simulink model "ROPOD_Control_WheelsRL_Code_GEN"  (R2020b)
settings: Solver=VariableStepAuto  StartTime=0.0  StopTime=10.0  RelTol=1e-3
values from neighbouring files (symbols this model uses):
  FFtheta_intia = 0    [init_model.m]
  FFxy_mass = 0*80    (= 0)    [init_model.m]
  I_fhz_ddelta_cntr = 0    [init_model.m]
  I_fhz_dtheta_cntr = 0.3    [init_model.m]
  I_fhz_dxdy_cntr = 0.25    [init_model.m]
  K_gain_ddelta_cntr = 0.2    [init_model.m]
  K_gain_dtheta_cntr = 150    [init_model.m]
  K_gain_dxdy_cntr = 200    [init_model.m]
  LL_wp_fhz_ddelta_cntr = 10    [init_model.m]
  LL_wp_fhz_dtheta_cntr = 20    [init_model.m]
  LL_wp_fhz_dxdy_cntr = 20    [init_model.m]
  LL_wz_fhz_ddelta_cntr = 2    [init_model.m]
  LL_wz_fhz_dtheta_cntr = 20    [init_model.m]
  LL_wz_fhz_dxdy_cntr = 20    [init_model.m]
  LPF_fhz_ddelta_cntr = 10    [init_model.m]
  LPF_fhz_ddelta_meas = 50    [init_model.m]
  LPF_fhz_dtheta_cntr = 100    [init_model.m]
  LPF_fhz_dvarphi_meas = 50    [init_model.m]
  LPF_fhz_dxdy_cntr = 100    [init_model.m]
  max_hw_tau = 7.0    (= 7)    [init_model.m]
  max_ropod_acc_theta = 1.6    [init_model.m]
  max_ropod_acc_xy = 2.0    (= 2)    [init_model.m]
  max_ropod_sw_force = 500    [init_model.m]
  max_ropod_sw_tau = 250    [init_model.m]
  max_ropod_vel_theta = 1.6    [init_model.m]
  max_ropod_vel_xy = 2.0    (= 2)    [init_model.m]
  max_sw_current = 10    [init_model.m]
  Nwheels = 4    [Jqwl_numeric_function.m]    (also in S_matrix.m; extract_kinmodel_parameters.m; init_model.m; tau_optimal_dist_vec_fun.m)
  pivot_offs_sws = [3.835 3.465 2.059 0.357]    [init_model.m]
  ropod_kinmodel_pv = struct2array(ropod_kinmodel_param)    [set_ropod_KinModparams.m]
  SW_COM1_ENABLE1 = hex2dec('0001')    [init_model.m]
  SW_COM1_ENABLE2 = hex2dec('0002')    [init_model.m]
  SW_COM1_MODE_TORQUE = bitshift(hex2dec('0000'),2)    [init_model.m]
  SW_COM1_MODE_VELOCITY = bitshift(hex2dec('0002'),2)    [init_model.m]
  SW_COM1_USE_TS = hex2dec('8000')    [init_model.m]
  Tinit = 0*Tslot    [init_model.m]
  Ts = 0.001    [init_model.m]
undefined symbols (not defined in the file or in its folder): AgentNumber, DiscIntNeverNeededParam, flock_FFtheta_friction, flock_FFxy_friction, I_fhz_dtheta_flock_cntr, I_fhz_dvarphi_cntr, I_fhz_dxdy_flock_cntr, K_gain_dtheta_flock_cntr, K_gain_dvarphi_cntr, K_gain_dxdy_flock_cntr, LL_wp_fhz_dtheta_flock_cntr, LL_wp_fhz_dvarphi_cntr, LL_wp_fhz_dxdy_flock_cntr, LL_wz_fhz_dtheta_flock_cntr, LL_wz_fhz_dvarphi_cntr, LL_wz_fhz_dxdy_flock_cntr, LPF_fhz_dtheta_flock_cntr, LPF_fhz_dvarphi_cntr, LPF_fhz_dxdy_flock_cntr, max_flock_acc_theta, max_flock_acc_xy, max_flock_vel_theta, max_flock_vel_xy, Nagents, ropod_position_inflock, sw_tau_2_current, Tsflck
libraries: simulink x62, pid_lib x60, cstblocks x54, dspsigops x24, SOEM_EtherCAT_Lib x5, dspnetwork x4
(part 9 of 11)

== system ROPOD_Control_WheelsRL_Code_GEN/RopodTorqueDistribution_/pivot damping cntr/Pivot controller/G_I_LL_LPF Controller4/Shapeit Lead-Lag (Tustin) ==
  In : Inport
  fz : Inport  Port=2
  fp : Inport  Port=3
  Add : Sum  Inputs=+-
  Constant1 : Constant
  Constant2 : Constant  Value=0
  Constant4 : Constant
  Divide : Product  Inputs=*/
  Divide1 : Product  Inputs=/*
  Gain1 : Gain  Gain=2*pi
  Gain2 : Gain  Gain=2*pi
  PID Controller3 : pid_lib/PID Controller  Controller=PID  Form=Parallel  TimeDomain=Discrete-time  UseExternalTs=off  SampleTime=Ts  IntegratorMethod=Trapezoidal  FilterMethod=Trapezoidal  ControllerParametersSource=external  P=0.4  I=0.4*2*pi*3  D=0  UseFilter=on  N=100  TunerSelectOption=Transfer Function Based (PID Tuner App)  InitialConditionSource=internal  InitialConditionForIntegrator=0  InitialConditionForFilter=0  DifferentiatorICPrevScaledInput=0  ExternalReset=none  TrackingMode=off  Kt=1  LimitOutput=off  SatLimitsSource=internal  UpperSaturationLimit=max_hw_tau  LowerSaturationLimit=-max_hw_tau  LinearizeAsGain=on  AntiWindupMode=clamping  Kb=1  POutMin=[]  POutMax=[]  IOutMin=[]  IOutMax=[]  DOutMin=[]  DOutMax=[]  NOutMin=[]  NOutMax=[]  SumOutMin=[]  SumOutMax=[]  SaturationOutMin=[]  SaturationOutMax=[]  PParamMin=[]  PParamMax=[]  IParamMin=[]  IParamMax=[]  DParamMin=[]  DParamMax=[]  NParamMin=[]  NParamMax=[]  KbParamMin=[]  KbParamMax=[]  KtParamMin=[]  KtParamMax=[]  KbOutMin=[]  KbOutMax=[]  KtOutMin=[]  KtOutMax=[]  IntegratorOutMin=[]  IntegratorOutMax=[]  FilterOutMin=[]  FilterOutMax=[]  SumI1OutMin=[]  SumI1OutMax=[]  SumI2OutMin=[]  SumI2OutMax=[]  SumI3OutMin=[]  SumI3OutMax=[]  SumI4OutMin=[]  SumI4OutMax=[]  SumDOutMin=[]  SumDOutMax=[]  DifferentiatorOutMin=[]  DifferentiatorOutMax=[]  FilterDiffOutCoefMin=[]  FilterDiffOutCoefMax=[]  ReciprocalOutMin=[]  ReciprocalOutMax=[]  SumDenOutMin=[]  SumDenOutMax=[]  SumNumOutMin=[]  SumNumOutMax=[]  DivideOutMin=[]  DivideOutMax=[]  UdiffTsProdOutMin=[]  UdiffTsProdOutMax=[]  NTsProdOutMin=[]  NTsProdOutMax=[]  UintegralTsProdOutMin=[]  UintegralTsProdOutMax=[]  UngainTsProdOutMin=[]  UngainTsProdOutMax=[]  IntegratorContinuousStateAttributes=''  IntegratorStateMustResolveToSignalObject=off  IntegratorRTWStateStorageClass=Auto  FilterContinuousStateAttributes=''  FilterStateMustResolveToSignalObject=off  FilterRTWStateStorageClass=Auto  ParallelPVariant=ExternalParameters  IdealPVariant=Disabled  IVariant=ExternalParameters  DVariant=ExternalParameters  IntegratorVariant=Discrete  SatVariant=Disabled  AWVariant=Passthrough  PCopyVariant=Disabled  TRVariant=Disabled  FdbkBlocksVariant=Forward  IdealPFdbkVariant=Disabled  SatFdbkVariant=Disabled  DerivativeFilterVariant=TrapezoidalFilter  NVariant=ExternalParameters  NCopyVariant=ExternalParameters  FilterICVariant=InternalICsFilter  IntegratorICVariant=InternalICs  ExternalResetVariant=Disabled  TRSumVariant=Passthrough  SumFdbkVariant=Disabled  SumVariant=Sum_PID  TsampFilterVariant=InternalTs  TsampNgainVariant=Passthrough  TsampIntegralVariant=Passthrough  ExternalSaturationOutDataTypeStr=Inherit: Same as second input
  Out : Outport  VectorParamsAs1DForOutWhenUnconnected=off
  wires:
  Constant4/1 -> PID Controller3/2
  In/1 -> PID Controller3/1
  PID Controller3/1 -> Out/1
  fz/1 -> Gain2/1
  fp/1 -> Gain1/1
  Gain1/1 -> PID Controller3/5, Divide/2
  Constant2/1 -> PID Controller3/3
  Gain2/1 -> Divide1/1, Divide/1
  Divide/1 -> Add/2
  Constant1/1 -> Add/1
  Add/1 -> Divide1/2
  Divide1/1 -> PID Controller3/4

== system ROPOD_Control_WheelsRL_Code_GEN/RopodTorqueDistribution_/wheel vel cntr/Wheels Velocity controller/G_I_LL_LPF Controller1/Shapeit Integrator (Tustin) ==
  In : Inport
  I_fhz : Inport  Port=2
  reset : Inport  Port=3
  Constant : Constant  Value=0
  Constant4 : Constant
  Constant5 : Constant  Value=0
  Gain2 : Gain  Gain=2*pi
  PID Controller3 : pid_lib/PID Controller  Controller=PID  Form=Parallel  TimeDomain=Discrete-time  UseExternalTs=off  SampleTime=Ts  IntegratorMethod=Trapezoidal  FilterMethod=Trapezoidal  ControllerParametersSource=external  P=0.4  I=0.4*2*pi*3  D=0  UseFilter=on  N=100  TunerSelectOption=Transfer Function Based (PID Tuner App)  InitialConditionSource=internal  InitialConditionForIntegrator=0  InitialConditionForFilter=0  DifferentiatorICPrevScaledInput=0  ExternalReset=level  TrackingMode=off  Kt=1  LimitOutput=on  SatLimitsSource=internal  UpperSaturationLimit=max_hw_tau  LowerSaturationLimit=-max_hw_tau  LinearizeAsGain=on  AntiWindupMode=clamping  Kb=1  POutMin=[]  POutMax=[]  IOutMin=[]  IOutMax=[]  DOutMin=[]  DOutMax=[]  NOutMin=[]  NOutMax=[]  SumOutMin=[]  SumOutMax=[]  SaturationOutMin=[]  SaturationOutMax=[]  PParamMin=[]  PParamMax=[]  IParamMin=[]  IParamMax=[]  DParamMin=[]  DParamMax=[]  NParamMin=[]  NParamMax=[]  KbParamMin=[]  KbParamMax=[]  KtParamMin=[]  KtParamMax=[]  KbOutMin=[]  KbOutMax=[]  KtOutMin=[]  KtOutMax=[]  IntegratorOutMin=[]  IntegratorOutMax=[]  FilterOutMin=[]  FilterOutMax=[]  SumI1OutMin=[]  SumI1OutMax=[]  SumI2OutMin=[]  SumI2OutMax=[]  SumI3OutMin=[]  SumI3OutMax=[]  SumI4OutMin=[]  SumI4OutMax=[]  SumDOutMin=[]  SumDOutMax=[]  DifferentiatorOutMin=[]  DifferentiatorOutMax=[]  FilterDiffOutCoefMin=[]  FilterDiffOutCoefMax=[]  ReciprocalOutMin=[]  ReciprocalOutMax=[]  SumDenOutMin=[]  SumDenOutMax=[]  SumNumOutMin=[]  SumNumOutMax=[]  DivideOutMin=[]  DivideOutMax=[]  UdiffTsProdOutMin=[]  UdiffTsProdOutMax=[]  NTsProdOutMin=[]  NTsProdOutMax=[]  UintegralTsProdOutMin=[]  UintegralTsProdOutMax=[]  UngainTsProdOutMin=[]  UngainTsProdOutMax=[]  IntegratorContinuousStateAttributes=''  IntegratorStateMustResolveToSignalObject=off  IntegratorRTWStateStorageClass=Auto  FilterContinuousStateAttributes=''  FilterStateMustResolveToSignalObject=off  FilterRTWStateStorageClass=Auto  ParallelPVariant=ExternalParameters  IdealPVariant=Disabled  IVariant=ExternalParameters  DVariant=ExternalParameters  IntegratorVariant=Discrete  SatVariant=Enabled  AWVariant=DiscClampingParallel  PCopyVariant=Disabled  TRVariant=Disabled  FdbkBlocksVariant=Feedback  IdealPFdbkVariant=Passthrough  SatFdbkVariant=Passthrough  DerivativeFilterVariant=TrapezoidalFilter  NVariant=ExternalParameters  NCopyVariant=ExternalParameters  FilterICVariant=InternalICsFilter  IntegratorICVariant=InternalICs  ExternalResetVariant=ExternalReset  TRSumVariant=Passthrough  SumFdbkVariant=Enabled  SumVariant=Sum_PID  TsampFilterVariant=InternalTs  TsampNgainVariant=Passthrough  TsampIntegralVariant=Passthrough  ExternalSaturationOutDataTypeStr=Inherit: Same as second input
  Product4 : Product
  Out : Outport  VectorParamsAs1DForOutWhenUnconnected=off
  wires:
  I_fhz/1 -> Product4/2
  Product4/1 -> Gain2/1
  reset/1 -> PID Controller3/6
  Gain2/1 -> PID Controller3/3
  PID Controller3/1 -> Out/1
  In/1 -> PID Controller3/1
  Constant4/1 -> Product4/1, PID Controller3/2
  Constant5/1 -> PID Controller3/5
  Constant/1 -> PID Controller3/4

== system ROPOD_Control_WheelsRL_Code_GEN/RopodTorqueDistribution_/wheel vel cntr/Wheels Velocity controller/G_I_LL_LPF Controller1/Shapeit Lead-Lag (Tustin) ==
  In : Inport
  fz : Inport  Port=2
  fp : Inport  Port=3
  Add : Sum  Inputs=+-
  Constant1 : Constant
  Constant2 : Constant  Value=0
  Constant4 : Constant
  Divide : Product  Inputs=*/
  Divide1 : Product  Inputs=/*
  Gain1 : Gain  Gain=2*pi
  Gain2 : Gain  Gain=2*pi
  PID Controller3 : pid_lib/PID Controller  Controller=PID  Form=Parallel  TimeDomain=Discrete-time  UseExternalTs=off  SampleTime=Ts  IntegratorMethod=Trapezoidal  FilterMethod=Trapezoidal  ControllerParametersSource=external  P=0.4  I=0.4*2*pi*3  D=0  UseFilter=on  N=100  TunerSelectOption=Transfer Function Based (PID Tuner App)  InitialConditionSource=internal  InitialConditionForIntegrator=0  InitialConditionForFilter=0  DifferentiatorICPrevScaledInput=0  ExternalReset=none  TrackingMode=off  Kt=1  LimitOutput=off  SatLimitsSource=internal  UpperSaturationLimit=max_hw_tau  LowerSaturationLimit=-max_hw_tau  LinearizeAsGain=on  AntiWindupMode=clamping  Kb=1  POutMin=[]  POutMax=[]  IOutMin=[]  IOutMax=[]  DOutMin=[]  DOutMax=[]  NOutMin=[]  NOutMax=[]  SumOutMin=[]  SumOutMax=[]  SaturationOutMin=[]  SaturationOutMax=[]  PParamMin=[]  PParamMax=[]  IParamMin=[]  IParamMax=[]  DParamMin=[]  DParamMax=[]  NParamMin=[]  NParamMax=[]  KbParamMin=[]  KbParamMax=[]  KtParamMin=[]  KtParamMax=[]  KbOutMin=[]  KbOutMax=[]  KtOutMin=[]  KtOutMax=[]  IntegratorOutMin=[]  IntegratorOutMax=[]  FilterOutMin=[]  FilterOutMax=[]  SumI1OutMin=[]  SumI1OutMax=[]  SumI2OutMin=[]  SumI2OutMax=[]  SumI3OutMin=[]  SumI3OutMax=[]  SumI4OutMin=[]  SumI4OutMax=[]  SumDOutMin=[]  SumDOutMax=[]  DifferentiatorOutMin=[]  DifferentiatorOutMax=[]  FilterDiffOutCoefMin=[]  FilterDiffOutCoefMax=[]  ReciprocalOutMin=[]  ReciprocalOutMax=[]  SumDenOutMin=[]  SumDenOutMax=[]  SumNumOutMin=[]  SumNumOutMax=[]  DivideOutMin=[]  DivideOutMax=[]  UdiffTsProdOutMin=[]  UdiffTsProdOutMax=[]  NTsProdOutMin=[]  NTsProdOutMax=[]  UintegralTsProdOutMin=[]  UintegralTsProdOutMax=[]  UngainTsProdOutMin=[]  UngainTsProdOutMax=[]  IntegratorContinuousStateAttributes=''  IntegratorStateMustResolveToSignalObject=off  IntegratorRTWStateStorageClass=Auto  FilterContinuousStateAttributes=''  FilterStateMustResolveToSignalObject=off  FilterRTWStateStorageClass=Auto  ParallelPVariant=ExternalParameters  IdealPVariant=Disabled  IVariant=ExternalParameters  DVariant=ExternalParameters  IntegratorVariant=Discrete  SatVariant=Disabled  AWVariant=Passthrough  PCopyVariant=Disabled  TRVariant=Disabled  FdbkBlocksVariant=Forward  IdealPFdbkVariant=Disabled  SatFdbkVariant=Disabled  DerivativeFilterVariant=TrapezoidalFilter  NVariant=ExternalParameters  NCopyVariant=ExternalParameters  FilterICVariant=InternalICsFilter  IntegratorICVariant=InternalICs  ExternalResetVariant=Disabled  TRSumVariant=Passthrough  SumFdbkVariant=Disabled  SumVariant=Sum_PID  TsampFilterVariant=InternalTs  TsampNgainVariant=Passthrough  TsampIntegralVariant=Passthrough  ExternalSaturationOutDataTypeStr=Inherit: Same as second input
  Out : Outport  VectorParamsAs1DForOutWhenUnconnected=off
  wires:
  Constant4/1 -> PID Controller3/2
  In/1 -> PID Controller3/1
  PID Controller3/1 -> Out/1
  fz/1 -> Gain2/1
  fp/1 -> Gain1/1
  Gain1/1 -> PID Controller3/5, Divide/2
  Constant2/1 -> PID Controller3/3
  Gain2/1 -> Divide1/1, Divide/1
  Divide/1 -> Add/2
  Constant1/1 -> Add/1
  Add/1 -> Divide1/2
  Divide1/1 -> PID Controller3/4

== system ROPOD_Control_WheelsRL_Code_GEN/RopodTorqueDistribution_/wheel vel cntr/Wheels Velocity controller/G_I_LL_LPF Controller2/Shapeit Integrator (Tustin) ==
  In : Inport
  I_fhz : Inport  Port=2
  reset : Inport  Port=3
  Constant : Constant  Value=0
  Constant4 : Constant
  Constant5 : Constant  Value=0
  Gain2 : Gain  Gain=2*pi
  PID Controller3 : pid_lib/PID Controller  Controller=PID  Form=Parallel  TimeDomain=Discrete-time  UseExternalTs=off  SampleTime=Ts  IntegratorMethod=Trapezoidal  FilterMethod=Trapezoidal  ControllerParametersSource=external  P=0.4  I=0.4*2*pi*3  D=0  UseFilter=on  N=100  TunerSelectOption=Transfer Function Based (PID Tuner App)  InitialConditionSource=internal  InitialConditionForIntegrator=0  InitialConditionForFilter=0  DifferentiatorICPrevScaledInput=0  ExternalReset=level  TrackingMode=off  Kt=1  LimitOutput=on  SatLimitsSource=internal  UpperSaturationLimit=max_hw_tau  LowerSaturationLimit=-max_hw_tau  LinearizeAsGain=on  AntiWindupMode=clamping  Kb=1  POutMin=[]  POutMax=[]  IOutMin=[]  IOutMax=[]  DOutMin=[]  DOutMax=[]  NOutMin=[]  NOutMax=[]  SumOutMin=[]  SumOutMax=[]  SaturationOutMin=[]  SaturationOutMax=[]  PParamMin=[]  PParamMax=[]  IParamMin=[]  IParamMax=[]  DParamMin=[]  DParamMax=[]  NParamMin=[]  NParamMax=[]  KbParamMin=[]  KbParamMax=[]  KtParamMin=[]  KtParamMax=[]  KbOutMin=[]  KbOutMax=[]  KtOutMin=[]  KtOutMax=[]  IntegratorOutMin=[]  IntegratorOutMax=[]  FilterOutMin=[]  FilterOutMax=[]  SumI1OutMin=[]  SumI1OutMax=[]  SumI2OutMin=[]  SumI2OutMax=[]  SumI3OutMin=[]  SumI3OutMax=[]  SumI4OutMin=[]  SumI4OutMax=[]  SumDOutMin=[]  SumDOutMax=[]  DifferentiatorOutMin=[]  DifferentiatorOutMax=[]  FilterDiffOutCoefMin=[]  FilterDiffOutCoefMax=[]  ReciprocalOutMin=[]  ReciprocalOutMax=[]  SumDenOutMin=[]  SumDenOutMax=[]  SumNumOutMin=[]  SumNumOutMax=[]  DivideOutMin=[]  DivideOutMax=[]  UdiffTsProdOutMin=[]  UdiffTsProdOutMax=[]  NTsProdOutMin=[]  NTsProdOutMax=[]  UintegralTsProdOutMin=[]  UintegralTsProdOutMax=[]  UngainTsProdOutMin=[]  UngainTsProdOutMax=[]  IntegratorContinuousStateAttributes=''  IntegratorStateMustResolveToSignalObject=off  IntegratorRTWStateStorageClass=Auto  FilterContinuousStateAttributes=''  FilterStateMustResolveToSignalObject=off  FilterRTWStateStorageClass=Auto  ParallelPVariant=ExternalParameters  IdealPVariant=Disabled  IVariant=ExternalParameters  DVariant=ExternalParameters  IntegratorVariant=Discrete  SatVariant=Enabled  AWVariant=DiscClampingParallel  PCopyVariant=Disabled  TRVariant=Disabled  FdbkBlocksVariant=Feedback  IdealPFdbkVariant=Passthrough  SatFdbkVariant=Passthrough  DerivativeFilterVariant=TrapezoidalFilter  NVariant=ExternalParameters  NCopyVariant=ExternalParameters  FilterICVariant=InternalICsFilter  IntegratorICVariant=InternalICs  ExternalResetVariant=ExternalReset  TRSumVariant=Passthrough  SumFdbkVariant=Enabled  SumVariant=Sum_PID  TsampFilterVariant=InternalTs  TsampNgainVariant=Passthrough  TsampIntegralVariant=Passthrough  ExternalSaturationOutDataTypeStr=Inherit: Same as second input
  Product4 : Product
  Out : Outport  VectorParamsAs1DForOutWhenUnconnected=off
  wires:
  I_fhz/1 -> Product4/2
  Product4/1 -> Gain2/1
  reset/1 -> PID Controller3/6
  Gain2/1 -> PID Controller3/3
  PID Controller3/1 -> Out/1
  In/1 -> PID Controller3/1
  Constant4/1 -> Product4/1, PID Controller3/2
  Constant5/1 -> PID Controller3/5
  Constant/1 -> PID Controller3/4

== system ROPOD_Control_WheelsRL_Code_GEN/RopodTorqueDistribution_/wheel vel cntr/Wheels Velocity controller/G_I_LL_LPF Controller2/Shapeit Lead-Lag (Tustin) ==
  In : Inport
  fz : Inport  Port=2
  fp : Inport  Port=3
  Add : Sum  Inputs=+-
  Constant1 : Constant
  Constant2 : Constant  Value=0
  Constant4 : Constant
  Divide : Product  Inputs=*/
  Divide1 : Product  Inputs=/*
  Gain1 : Gain  Gain=2*pi
  Gain2 : Gain  Gain=2*pi
  PID Controller3 : pid_lib/PID Controller  Controller=PID  Form=Parallel  TimeDomain=Discrete-time  UseExternalTs=off  SampleTime=Ts  IntegratorMethod=Trapezoidal  FilterMethod=Trapezoidal  ControllerParametersSource=external  P=0.4  I=0.4*2*pi*3  D=0  UseFilter=on  N=100  TunerSelectOption=Transfer Function Based (PID Tuner App)  InitialConditionSource=internal  InitialConditionForIntegrator=0  InitialConditionForFilter=0  DifferentiatorICPrevScaledInput=0  ExternalReset=none  TrackingMode=off  Kt=1  LimitOutput=off  SatLimitsSource=internal  UpperSaturationLimit=max_hw_tau  LowerSaturationLimit=-max_hw_tau  LinearizeAsGain=on  AntiWindupMode=clamping  Kb=1  POutMin=[]  POutMax=[]  IOutMin=[]  IOutMax=[]  DOutMin=[]  DOutMax=[]  NOutMin=[]  NOutMax=[]  SumOutMin=[]  SumOutMax=[]  SaturationOutMin=[]  SaturationOutMax=[]  PParamMin=[]  PParamMax=[]  IParamMin=[]  IParamMax=[]  DParamMin=[]  DParamMax=[]  NParamMin=[]  NParamMax=[]  KbParamMin=[]  KbParamMax=[]  KtParamMin=[]  KtParamMax=[]  KbOutMin=[]  KbOutMax=[]  KtOutMin=[]  KtOutMax=[]  IntegratorOutMin=[]  IntegratorOutMax=[]  FilterOutMin=[]  FilterOutMax=[]  SumI1OutMin=[]  SumI1OutMax=[]  SumI2OutMin=[]  SumI2OutMax=[]  SumI3OutMin=[]  SumI3OutMax=[]  SumI4OutMin=[]  SumI4OutMax=[]  SumDOutMin=[]  SumDOutMax=[]  DifferentiatorOutMin=[]  DifferentiatorOutMax=[]  FilterDiffOutCoefMin=[]  FilterDiffOutCoefMax=[]  ReciprocalOutMin=[]  ReciprocalOutMax=[]  SumDenOutMin=[]  SumDenOutMax=[]  SumNumOutMin=[]  SumNumOutMax=[]  DivideOutMin=[]  DivideOutMax=[]  UdiffTsProdOutMin=[]  UdiffTsProdOutMax=[]  NTsProdOutMin=[]  NTsProdOutMax=[]  UintegralTsProdOutMin=[]  UintegralTsProdOutMax=[]  UngainTsProdOutMin=[]  UngainTsProdOutMax=[]  IntegratorContinuousStateAttributes=''  IntegratorStateMustResolveToSignalObject=off  IntegratorRTWStateStorageClass=Auto  FilterContinuousStateAttributes=''  FilterStateMustResolveToSignalObject=off  FilterRTWStateStorageClass=Auto  ParallelPVariant=ExternalParameters  IdealPVariant=Disabled  IVariant=ExternalParameters  DVariant=ExternalParameters  IntegratorVariant=Discrete  SatVariant=Disabled  AWVariant=Passthrough  PCopyVariant=Disabled  TRVariant=Disabled  FdbkBlocksVariant=Forward  IdealPFdbkVariant=Disabled  SatFdbkVariant=Disabled  DerivativeFilterVariant=TrapezoidalFilter  NVariant=ExternalParameters  NCopyVariant=ExternalParameters  FilterICVariant=InternalICsFilter  IntegratorICVariant=InternalICs  ExternalResetVariant=Disabled  TRSumVariant=Passthrough  SumFdbkVariant=Disabled  SumVariant=Sum_PID  TsampFilterVariant=InternalTs  TsampNgainVariant=Passthrough  TsampIntegralVariant=Passthrough  ExternalSaturationOutDataTypeStr=Inherit: Same as second input
  Out : Outport  VectorParamsAs1DForOutWhenUnconnected=off
  wires:
  Constant4/1 -> PID Controller3/2
  In/1 -> PID Controller3/1
  PID Controller3/1 -> Out/1
  fz/1 -> Gain2/1
  fp/1 -> Gain1/1
  Gain1/1 -> PID Controller3/5, Divide/2
  Constant2/1 -> PID Controller3/3
  Gain2/1 -> Divide1/1, Divide/1
  Divide/1 -> Add/2
  Constant1/1 -> Add/1
  Add/1 -> Divide1/2
  Divide1/1 -> PID Controller3/4

== system ROPOD_Control_WheelsRL_Code_GEN/RopodTorqueDistribution_/wheel vel cntr/Wheels Velocity controller/G_I_LL_LPF Controller3/Shapeit Integrator (Tustin) ==
  In : Inport
  I_fhz : Inport  Port=2
  reset : Inport  Port=3
  Constant : Constant  Value=0
  Constant4 : Constant
  Constant5 : Constant  Value=0
  Gain2 : Gain  Gain=2*pi
  PID Controller3 : pid_lib/PID Controller  Controller=PID  Form=Parallel  TimeDomain=Discrete-time  UseExternalTs=off  SampleTime=Ts  IntegratorMethod=Trapezoidal  FilterMethod=Trapezoidal  ControllerParametersSource=external  P=0.4  I=0.4*2*pi*3  D=0  UseFilter=on  N=100  TunerSelectOption=Transfer Function Based (PID Tuner App)  InitialConditionSource=internal  InitialConditionForIntegrator=0  InitialConditionForFilter=0  DifferentiatorICPrevScaledInput=0  ExternalReset=level  TrackingMode=off  Kt=1  LimitOutput=on  SatLimitsSource=internal  UpperSaturationLimit=max_hw_tau  LowerSaturationLimit=-max_hw_tau  LinearizeAsGain=on  AntiWindupMode=clamping  Kb=1  POutMin=[]  POutMax=[]  IOutMin=[]  IOutMax=[]  DOutMin=[]  DOutMax=[]  NOutMin=[]  NOutMax=[]  SumOutMin=[]  SumOutMax=[]  SaturationOutMin=[]  SaturationOutMax=[]  PParamMin=[]  PParamMax=[]  IParamMin=[]  IParamMax=[]  DParamMin=[]  DParamMax=[]  NParamMin=[]  NParamMax=[]  KbParamMin=[]  KbParamMax=[]  KtParamMin=[]  KtParamMax=[]  KbOutMin=[]  KbOutMax=[]  KtOutMin=[]  KtOutMax=[]  IntegratorOutMin=[]  IntegratorOutMax=[]  FilterOutMin=[]  FilterOutMax=[]  SumI1OutMin=[]  SumI1OutMax=[]  SumI2OutMin=[]  SumI2OutMax=[]  SumI3OutMin=[]  SumI3OutMax=[]  SumI4OutMin=[]  SumI4OutMax=[]  SumDOutMin=[]  SumDOutMax=[]  DifferentiatorOutMin=[]  DifferentiatorOutMax=[]  FilterDiffOutCoefMin=[]  FilterDiffOutCoefMax=[]  ReciprocalOutMin=[]  ReciprocalOutMax=[]  SumDenOutMin=[]  SumDenOutMax=[]  SumNumOutMin=[]  SumNumOutMax=[]  DivideOutMin=[]  DivideOutMax=[]  UdiffTsProdOutMin=[]  UdiffTsProdOutMax=[]  NTsProdOutMin=[]  NTsProdOutMax=[]  UintegralTsProdOutMin=[]  UintegralTsProdOutMax=[]  UngainTsProdOutMin=[]  UngainTsProdOutMax=[]  IntegratorContinuousStateAttributes=''  IntegratorStateMustResolveToSignalObject=off  IntegratorRTWStateStorageClass=Auto  FilterContinuousStateAttributes=''  FilterStateMustResolveToSignalObject=off  FilterRTWStateStorageClass=Auto  ParallelPVariant=ExternalParameters  IdealPVariant=Disabled  IVariant=ExternalParameters  DVariant=ExternalParameters  IntegratorVariant=Discrete  SatVariant=Enabled  AWVariant=DiscClampingParallel  PCopyVariant=Disabled  TRVariant=Disabled  FdbkBlocksVariant=Feedback  IdealPFdbkVariant=Passthrough  SatFdbkVariant=Passthrough  DerivativeFilterVariant=TrapezoidalFilter  NVariant=ExternalParameters  NCopyVariant=ExternalParameters  FilterICVariant=InternalICsFilter  IntegratorICVariant=InternalICs  ExternalResetVariant=ExternalReset  TRSumVariant=Passthrough  SumFdbkVariant=Enabled  SumVariant=Sum_PID  TsampFilterVariant=InternalTs  TsampNgainVariant=Passthrough  TsampIntegralVariant=Passthrough  ExternalSaturationOutDataTypeStr=Inherit: Same as second input
  Product4 : Product
  Out : Outport  VectorParamsAs1DForOutWhenUnconnected=off
  wires:
  Constant/1 -> PID Controller3/4
  Constant5/1 -> PID Controller3/5
  Constant4/1 -> PID Controller3/2, Product4/1
  In/1 -> PID Controller3/1
  PID Controller3/1 -> Out/1
  Gain2/1 -> PID Controller3/3
  reset/1 -> PID Controller3/6
  Product4/1 -> Gain2/1
  I_fhz/1 -> Product4/2

== system ROPOD_Control_WheelsRL_Code_GEN/RopodTorqueDistribution_/wheel vel cntr/Wheels Velocity controller/G_I_LL_LPF Controller3/Shapeit Lead-Lag (Tustin) ==
  In : Inport
  fz : Inport  Port=2
  fp : Inport  Port=3
  Add : Sum  Inputs=+-
  Constant1 : Constant
  Constant2 : Constant  Value=0
  Constant4 : Constant
  Divide : Product  Inputs=*/
  Divide1 : Product  Inputs=/*
  Gain1 : Gain  Gain=2*pi
  Gain2 : Gain  Gain=2*pi
  PID Controller3 : pid_lib/PID Controller  Controller=PID  Form=Parallel  TimeDomain=Discrete-time  UseExternalTs=off  SampleTime=Ts  IntegratorMethod=Trapezoidal  FilterMethod=Trapezoidal  ControllerParametersSource=external  P=0.4  I=0.4*2*pi*3  D=0  UseFilter=on  N=100  TunerSelectOption=Transfer Function Based (PID Tuner App)  InitialConditionSource=internal  InitialConditionForIntegrator=0  InitialConditionForFilter=0  DifferentiatorICPrevScaledInput=0  ExternalReset=none  TrackingMode=off  Kt=1  LimitOutput=off  SatLimitsSource=internal  UpperSaturationLimit=max_hw_tau  LowerSaturationLimit=-max_hw_tau  LinearizeAsGain=on  AntiWindupMode=clamping  Kb=1  POutMin=[]  POutMax=[]  IOutMin=[]  IOutMax=[]  DOutMin=[]  DOutMax=[]  NOutMin=[]  NOutMax=[]  SumOutMin=[]  SumOutMax=[]  SaturationOutMin=[]  SaturationOutMax=[]  PParamMin=[]  PParamMax=[]  IParamMin=[]  IParamMax=[]  DParamMin=[]  DParamMax=[]  NParamMin=[]  NParamMax=[]  KbParamMin=[]  KbParamMax=[]  KtParamMin=[]  KtParamMax=[]  KbOutMin=[]  KbOutMax=[]  KtOutMin=[]  KtOutMax=[]  IntegratorOutMin=[]  IntegratorOutMax=[]  FilterOutMin=[]  FilterOutMax=[]  SumI1OutMin=[]  SumI1OutMax=[]  SumI2OutMin=[]  SumI2OutMax=[]  SumI3OutMin=[]  SumI3OutMax=[]  SumI4OutMin=[]  SumI4OutMax=[]  SumDOutMin=[]  SumDOutMax=[]  DifferentiatorOutMin=[]  DifferentiatorOutMax=[]  FilterDiffOutCoefMin=[]  FilterDiffOutCoefMax=[]  ReciprocalOutMin=[]  ReciprocalOutMax=[]  SumDenOutMin=[]  SumDenOutMax=[]  SumNumOutMin=[]  SumNumOutMax=[]  DivideOutMin=[]  DivideOutMax=[]  UdiffTsProdOutMin=[]  UdiffTsProdOutMax=[]  NTsProdOutMin=[]  NTsProdOutMax=[]  UintegralTsProdOutMin=[]  UintegralTsProdOutMax=[]  UngainTsProdOutMin=[]  UngainTsProdOutMax=[]  IntegratorContinuousStateAttributes=''  IntegratorStateMustResolveToSignalObject=off  IntegratorRTWStateStorageClass=Auto  FilterContinuousStateAttributes=''  FilterStateMustResolveToSignalObject=off  FilterRTWStateStorageClass=Auto  ParallelPVariant=ExternalParameters  IdealPVariant=Disabled  IVariant=ExternalParameters  DVariant=ExternalParameters  IntegratorVariant=Discrete  SatVariant=Disabled  AWVariant=Passthrough  PCopyVariant=Disabled  TRVariant=Disabled  FdbkBlocksVariant=Forward  IdealPFdbkVariant=Disabled  SatFdbkVariant=Disabled  DerivativeFilterVariant=TrapezoidalFilter  NVariant=ExternalParameters  NCopyVariant=ExternalParameters  FilterICVariant=InternalICsFilter  IntegratorICVariant=InternalICs  ExternalResetVariant=Disabled  TRSumVariant=Passthrough  SumFdbkVariant=Disabled  SumVariant=Sum_PID  TsampFilterVariant=InternalTs  TsampNgainVariant=Passthrough  TsampIntegralVariant=Passthrough  ExternalSaturationOutDataTypeStr=Inherit: Same as second input
  Out : Outport  VectorParamsAs1DForOutWhenUnconnected=off
  wires:
  Divide1/1 -> PID Controller3/4
  Add/1 -> Divide1/2
  Constant1/1 -> Add/1
  Divide/1 -> Add/2
  Gain2/1 -> Divide/1, Divide1/1
  Constant2/1 -> PID Controller3/3
  Gain1/1 -> Divide/2, PID Controller3/5
  fp/1 -> Gain1/1
  fz/1 -> Gain2/1
  PID Controller3/1 -> Out/1
  In/1 -> PID Controller3/1
  Constant4/1 -> PID Controller3/2

== system ROPOD_Control_WheelsRL_Code_GEN/RopodTorqueDistribution_/wheel vel cntr/Wheels Velocity controller/G_I_LL_LPF Controller4/Shapeit Integrator (Tustin) ==
  In : Inport
  I_fhz : Inport  Port=2
  reset : Inport  Port=3
  Constant : Constant  Value=0
  Constant4 : Constant
  Constant5 : Constant  Value=0
  Gain2 : Gain  Gain=2*pi
  PID Controller3 : pid_lib/PID Controller  Controller=PID  Form=Parallel  TimeDomain=Discrete-time  UseExternalTs=off  SampleTime=Ts  IntegratorMethod=Trapezoidal  FilterMethod=Trapezoidal  ControllerParametersSource=external  P=0.4  I=0.4*2*pi*3  D=0  UseFilter=on  N=100  TunerSelectOption=Transfer Function Based (PID Tuner App)  InitialConditionSource=internal  InitialConditionForIntegrator=0  InitialConditionForFilter=0  DifferentiatorICPrevScaledInput=0  ExternalReset=level  TrackingMode=off  Kt=1  LimitOutput=on  SatLimitsSource=internal  UpperSaturationLimit=max_hw_tau  LowerSaturationLimit=-max_hw_tau  LinearizeAsGain=on  AntiWindupMode=clamping  Kb=1  POutMin=[]  POutMax=[]  IOutMin=[]  IOutMax=[]  DOutMin=[]  DOutMax=[]  NOutMin=[]  NOutMax=[]  SumOutMin=[]  SumOutMax=[]  SaturationOutMin=[]  SaturationOutMax=[]  PParamMin=[]  PParamMax=[]  IParamMin=[]  IParamMax=[]  DParamMin=[]  DParamMax=[]  NParamMin=[]  NParamMax=[]  KbParamMin=[]  KbParamMax=[]  KtParamMin=[]  KtParamMax=[]  KbOutMin=[]  KbOutMax=[]  KtOutMin=[]  KtOutMax=[]  IntegratorOutMin=[]  IntegratorOutMax=[]  FilterOutMin=[]  FilterOutMax=[]  SumI1OutMin=[]  SumI1OutMax=[]  SumI2OutMin=[]  SumI2OutMax=[]  SumI3OutMin=[]  SumI3OutMax=[]  SumI4OutMin=[]  SumI4OutMax=[]  SumDOutMin=[]  SumDOutMax=[]  DifferentiatorOutMin=[]  DifferentiatorOutMax=[]  FilterDiffOutCoefMin=[]  FilterDiffOutCoefMax=[]  ReciprocalOutMin=[]  ReciprocalOutMax=[]  SumDenOutMin=[]  SumDenOutMax=[]  SumNumOutMin=[]  SumNumOutMax=[]  DivideOutMin=[]  DivideOutMax=[]  UdiffTsProdOutMin=[]  UdiffTsProdOutMax=[]  NTsProdOutMin=[]  NTsProdOutMax=[]  UintegralTsProdOutMin=[]  UintegralTsProdOutMax=[]  UngainTsProdOutMin=[]  UngainTsProdOutMax=[]  IntegratorContinuousStateAttributes=''  IntegratorStateMustResolveToSignalObject=off  IntegratorRTWStateStorageClass=Auto  FilterContinuousStateAttributes=''  FilterStateMustResolveToSignalObject=off  FilterRTWStateStorageClass=Auto  ParallelPVariant=ExternalParameters  IdealPVariant=Disabled  IVariant=ExternalParameters  DVariant=ExternalParameters  IntegratorVariant=Discrete  SatVariant=Enabled  AWVariant=DiscClampingParallel  PCopyVariant=Disabled  TRVariant=Disabled  FdbkBlocksVariant=Feedback  IdealPFdbkVariant=Passthrough  SatFdbkVariant=Passthrough  DerivativeFilterVariant=TrapezoidalFilter  NVariant=ExternalParameters  NCopyVariant=ExternalParameters  FilterICVariant=InternalICsFilter  IntegratorICVariant=InternalICs  ExternalResetVariant=ExternalReset  TRSumVariant=Passthrough  SumFdbkVariant=Enabled  SumVariant=Sum_PID  TsampFilterVariant=InternalTs  TsampNgainVariant=Passthrough  TsampIntegralVariant=Passthrough  ExternalSaturationOutDataTypeStr=Inherit: Same as second input
  Product4 : Product
  Out : Outport  VectorParamsAs1DForOutWhenUnconnected=off
  wires:
  I_fhz/1 -> Product4/2
  Product4/1 -> Gain2/1
  reset/1 -> PID Controller3/6
  Gain2/1 -> PID Controller3/3
  PID Controller3/1 -> Out/1
  In/1 -> PID Controller3/1
  Constant4/1 -> Product4/1, PID Controller3/2
  Constant5/1 -> PID Controller3/5
  Constant/1 -> PID Controller3/4

== system ROPOD_Control_WheelsRL_Code_GEN/RopodTorqueDistribution_/wheel vel cntr/Wheels Velocity controller/G_I_LL_LPF Controller4/Shapeit Lead-Lag (Tustin) ==
  In : Inport
  fz : Inport  Port=2
  fp : Inport  Port=3
  Add : Sum  Inputs=+-
  Constant1 : Constant
  Constant2 : Constant  Value=0
  Constant4 : Constant
  Divide : Product  Inputs=*/
  Divide1 : Product  Inputs=/*
  Gain1 : Gain  Gain=2*pi
  Gain2 : Gain  Gain=2*pi
  PID Controller3 : pid_lib/PID Controller  Controller=PID  Form=Parallel  TimeDomain=Discrete-time  UseExternalTs=off  SampleTime=Ts  IntegratorMethod=Trapezoidal  FilterMethod=Trapezoidal  ControllerParametersSource=external  P=0.4  I=0.4*2*pi*3  D=0  UseFilter=on  N=100  TunerSelectOption=Transfer Function Based (PID Tuner App)  InitialConditionSource=internal  InitialConditionForIntegrator=0  InitialConditionForFilter=0  DifferentiatorICPrevScaledInput=0  ExternalReset=none  TrackingMode=off  Kt=1  LimitOutput=off  SatLimitsSource=internal  UpperSaturationLimit=max_hw_tau  LowerSaturationLimit=-max_hw_tau  LinearizeAsGain=on  AntiWindupMode=clamping  Kb=1  POutMin=[]  POutMax=[]  IOutMin=[]  IOutMax=[]  DOutMin=[]  DOutMax=[]  NOutMin=[]  NOutMax=[]  SumOutMin=[]  SumOutMax=[]  SaturationOutMin=[]  SaturationOutMax=[]  PParamMin=[]  PParamMax=[]  IParamMin=[]  IParamMax=[]  DParamMin=[]  DParamMax=[]  NParamMin=[]  NParamMax=[]  KbParamMin=[]  KbParamMax=[]  KtParamMin=[]  KtParamMax=[]  KbOutMin=[]  KbOutMax=[]  KtOutMin=[]  KtOutMax=[]  IntegratorOutMin=[]  IntegratorOutMax=[]  FilterOutMin=[]  FilterOutMax=[]  SumI1OutMin=[]  SumI1OutMax=[]  SumI2OutMin=[]  SumI2OutMax=[]  SumI3OutMin=[]  SumI3OutMax=[]  SumI4OutMin=[]  SumI4OutMax=[]  SumDOutMin=[]  SumDOutMax=[]  DifferentiatorOutMin=[]  DifferentiatorOutMax=[]  FilterDiffOutCoefMin=[]  FilterDiffOutCoefMax=[]  ReciprocalOutMin=[]  ReciprocalOutMax=[]  SumDenOutMin=[]  SumDenOutMax=[]  SumNumOutMin=[]  SumNumOutMax=[]  DivideOutMin=[]  DivideOutMax=[]  UdiffTsProdOutMin=[]  UdiffTsProdOutMax=[]  NTsProdOutMin=[]  NTsProdOutMax=[]  UintegralTsProdOutMin=[]  UintegralTsProdOutMax=[]  UngainTsProdOutMin=[]  UngainTsProdOutMax=[]  IntegratorContinuousStateAttributes=''  IntegratorStateMustResolveToSignalObject=off  IntegratorRTWStateStorageClass=Auto  FilterContinuousStateAttributes=''  FilterStateMustResolveToSignalObject=off  FilterRTWStateStorageClass=Auto  ParallelPVariant=ExternalParameters  IdealPVariant=Disabled  IVariant=ExternalParameters  DVariant=ExternalParameters  IntegratorVariant=Discrete  SatVariant=Disabled  AWVariant=Passthrough  PCopyVariant=Disabled  TRVariant=Disabled  FdbkBlocksVariant=Forward  IdealPFdbkVariant=Disabled  SatFdbkVariant=Disabled  DerivativeFilterVariant=TrapezoidalFilter  NVariant=ExternalParameters  NCopyVariant=ExternalParameters  FilterICVariant=InternalICsFilter  IntegratorICVariant=InternalICs  ExternalResetVariant=Disabled  TRSumVariant=Passthrough  SumFdbkVariant=Disabled  SumVariant=Sum_PID  TsampFilterVariant=InternalTs  TsampNgainVariant=Passthrough  TsampIntegralVariant=Passthrough  ExternalSaturationOutDataTypeStr=Inherit: Same as second input
  Out : Outport  VectorParamsAs1DForOutWhenUnconnected=off
  wires:
  Constant4/1 -> PID Controller3/2
  In/1 -> PID Controller3/1
  PID Controller3/1 -> Out/1
  fz/1 -> Gain2/1
  fp/1 -> Gain1/1
  Gain1/1 -> PID Controller3/5, Divide/2
  Constant2/1 -> PID Controller3/3
  Gain2/1 -> Divide1/1, Divide/1
  Divide/1 -> Add/2
  Constant1/1 -> Add/1
  Add/1 -> Divide1/2
  Divide1/1 -> PID Controller3/4

== system ROPOD_Control_WheelsRL_Code_GEN/RopodTorqueDistribution_/wheel vel cntr/Wheels Velocity controller/G_I_LL_LPF Controller5/Shapeit Integrator (Tustin) ==
  In : Inport
  I_fhz : Inport  Port=2
  reset : Inport  Port=3
  Constant : Constant  Value=0
  Constant4 : Constant
  Constant5 : Constant  Value=0
  Gain2 : Gain  Gain=2*pi
  PID Controller3 : pid_lib/PID Controller  Controller=PID  Form=Parallel  TimeDomain=Discrete-time  UseExternalTs=off  SampleTime=Ts  IntegratorMethod=Trapezoidal  FilterMethod=Trapezoidal  ControllerParametersSource=external  P=0.4  I=0.4*2*pi*3  D=0  UseFilter=on  N=100  TunerSelectOption=Transfer Function Based (PID Tuner App)  InitialConditionSource=internal  InitialConditionForIntegrator=0  InitialConditionForFilter=0  DifferentiatorICPrevScaledInput=0  ExternalReset=level  TrackingMode=off  Kt=1  LimitOutput=on  SatLimitsSource=internal  UpperSaturationLimit=max_hw_tau  LowerSaturationLimit=-max_hw_tau  LinearizeAsGain=on  AntiWindupMode=clamping  Kb=1  POutMin=[]  POutMax=[]  IOutMin=[]  IOutMax=[]  DOutMin=[]  DOutMax=[]  NOutMin=[]  NOutMax=[]  SumOutMin=[]  SumOutMax=[]  SaturationOutMin=[]  SaturationOutMax=[]  PParamMin=[]  PParamMax=[]  IParamMin=[]  IParamMax=[]  DParamMin=[]  DParamMax=[]  NParamMin=[]  NParamMax=[]  KbParamMin=[]  KbParamMax=[]  KtParamMin=[]  KtParamMax=[]  KbOutMin=[]  KbOutMax=[]  KtOutMin=[]  KtOutMax=[]  IntegratorOutMin=[]  IntegratorOutMax=[]  FilterOutMin=[]  FilterOutMax=[]  SumI1OutMin=[]  SumI1OutMax=[]  SumI2OutMin=[]  SumI2OutMax=[]  SumI3OutMin=[]  SumI3OutMax=[]  SumI4OutMin=[]  SumI4OutMax=[]  SumDOutMin=[]  SumDOutMax=[]  DifferentiatorOutMin=[]  DifferentiatorOutMax=[]  FilterDiffOutCoefMin=[]  FilterDiffOutCoefMax=[]  ReciprocalOutMin=[]  ReciprocalOutMax=[]  SumDenOutMin=[]  SumDenOutMax=[]  SumNumOutMin=[]  SumNumOutMax=[]  DivideOutMin=[]  DivideOutMax=[]  UdiffTsProdOutMin=[]  UdiffTsProdOutMax=[]  NTsProdOutMin=[]  NTsProdOutMax=[]  UintegralTsProdOutMin=[]  UintegralTsProdOutMax=[]  UngainTsProdOutMin=[]  UngainTsProdOutMax=[]  IntegratorContinuousStateAttributes=''  IntegratorStateMustResolveToSignalObject=off  IntegratorRTWStateStorageClass=Auto  FilterContinuousStateAttributes=''  FilterStateMustResolveToSignalObject=off  FilterRTWStateStorageClass=Auto  ParallelPVariant=ExternalParameters  IdealPVariant=Disabled  IVariant=ExternalParameters  DVariant=ExternalParameters  IntegratorVariant=Discrete  SatVariant=Enabled  AWVariant=DiscClampingParallel  PCopyVariant=Disabled  TRVariant=Disabled  FdbkBlocksVariant=Feedback  IdealPFdbkVariant=Passthrough  SatFdbkVariant=Passthrough  DerivativeFilterVariant=TrapezoidalFilter  NVariant=ExternalParameters  NCopyVariant=ExternalParameters  FilterICVariant=InternalICsFilter  IntegratorICVariant=InternalICs  ExternalResetVariant=ExternalReset  TRSumVariant=Passthrough  SumFdbkVariant=Enabled  SumVariant=Sum_PID  TsampFilterVariant=InternalTs  TsampNgainVariant=Passthrough  TsampIntegralVariant=Passthrough  ExternalSaturationOutDataTypeStr=Inherit: Same as second input
  Product4 : Product
  Out : Outport  VectorParamsAs1DForOutWhenUnconnected=off
  wires:
  Constant/1 -> PID Controller3/4
  Constant5/1 -> PID Controller3/5
  Constant4/1 -> PID Controller3/2, Product4/1
  In/1 -> PID Controller3/1
  PID Controller3/1 -> Out/1
  Gain2/1 -> PID Controller3/3
  reset/1 -> PID Controller3/6
  Product4/1 -> Gain2/1
  I_fhz/1 -> Product4/2

== system ROPOD_Control_WheelsRL_Code_GEN/RopodTorqueDistribution_/wheel vel cntr/Wheels Velocity controller/G_I_LL_LPF Controller5/Shapeit Lead-Lag (Tustin) ==
  In : Inport
  fz : Inport  Port=2
  fp : Inport  Port=3
  Add : Sum  Inputs=+-
  Constant1 : Constant
  Constant2 : Constant  Value=0
  Constant4 : Constant
  Divide : Product  Inputs=*/
  Divide1 : Product  Inputs=/*
  Gain1 : Gain  Gain=2*pi
  Gain2 : Gain  Gain=2*pi
  PID Controller3 : pid_lib/PID Controller  Controller=PID  Form=Parallel  TimeDomain=Discrete-time  UseExternalTs=off  SampleTime=Ts  IntegratorMethod=Trapezoidal  FilterMethod=Trapezoidal  ControllerParametersSource=external  P=0.4  I=0.4*2*pi*3  D=0  UseFilter=on  N=100  TunerSelectOption=Transfer Function Based (PID Tuner App)  InitialConditionSource=internal  InitialConditionForIntegrator=0  InitialConditionForFilter=0  DifferentiatorICPrevScaledInput=0  ExternalReset=none  TrackingMode=off  Kt=1  LimitOutput=off  SatLimitsSource=internal  UpperSaturationLimit=max_hw_tau  LowerSaturationLimit=-max_hw_tau  LinearizeAsGain=on  AntiWindupMode=clamping  Kb=1  POutMin=[]  POutMax=[]  IOutMin=[]  IOutMax=[]  DOutMin=[]  DOutMax=[]  NOutMin=[]  NOutMax=[]  SumOutMin=[]  SumOutMax=[]  SaturationOutMin=[]  SaturationOutMax=[]  PParamMin=[]  PParamMax=[]  IParamMin=[]  IParamMax=[]  DParamMin=[]  DParamMax=[]  NParamMin=[]  NParamMax=[]  KbParamMin=[]  KbParamMax=[]  KtParamMin=[]  KtParamMax=[]  KbOutMin=[]  KbOutMax=[]  KtOutMin=[]  KtOutMax=[]  IntegratorOutMin=[]  IntegratorOutMax=[]  FilterOutMin=[]  FilterOutMax=[]  SumI1OutMin=[]  SumI1OutMax=[]  SumI2OutMin=[]  SumI2OutMax=[]  SumI3OutMin=[]  SumI3OutMax=[]  SumI4OutMin=[]  SumI4OutMax=[]  SumDOutMin=[]  SumDOutMax=[]  DifferentiatorOutMin=[]  DifferentiatorOutMax=[]  FilterDiffOutCoefMin=[]  FilterDiffOutCoefMax=[]  ReciprocalOutMin=[]  ReciprocalOutMax=[]  SumDenOutMin=[]  SumDenOutMax=[]  SumNumOutMin=[]  SumNumOutMax=[]  DivideOutMin=[]  DivideOutMax=[]  UdiffTsProdOutMin=[]  UdiffTsProdOutMax=[]  NTsProdOutMin=[]  NTsProdOutMax=[]  UintegralTsProdOutMin=[]  UintegralTsProdOutMax=[]  UngainTsProdOutMin=[]  UngainTsProdOutMax=[]  IntegratorContinuousStateAttributes=''  IntegratorStateMustResolveToSignalObject=off  IntegratorRTWStateStorageClass=Auto  FilterContinuousStateAttributes=''  FilterStateMustResolveToSignalObject=off  FilterRTWStateStorageClass=Auto  ParallelPVariant=ExternalParameters  IdealPVariant=Disabled  IVariant=ExternalParameters  DVariant=ExternalParameters  IntegratorVariant=Discrete  SatVariant=Disabled  AWVariant=Passthrough  PCopyVariant=Disabled  TRVariant=Disabled  FdbkBlocksVariant=Forward  IdealPFdbkVariant=Disabled  SatFdbkVariant=Disabled  DerivativeFilterVariant=TrapezoidalFilter  NVariant=ExternalParameters  NCopyVariant=ExternalParameters  FilterICVariant=InternalICsFilter  IntegratorICVariant=InternalICs  ExternalResetVariant=Disabled  TRSumVariant=Passthrough  SumFdbkVariant=Disabled  SumVariant=Sum_PID  TsampFilterVariant=InternalTs  TsampNgainVariant=Passthrough  TsampIntegralVariant=Passthrough  ExternalSaturationOutDataTypeStr=Inherit: Same as second input
  Out : Outport  VectorParamsAs1DForOutWhenUnconnected=off
  wires:
  Divide1/1 -> PID Controller3/4
  Add/1 -> Divide1/2
  Constant1/1 -> Add/1
  Divide/1 -> Add/2
  Gain2/1 -> Divide/1, Divide1/1
  Constant2/1 -> PID Controller3/3
  Gain1/1 -> Divide/2, PID Controller3/5
  fp/1 -> Gain1/1
  fz/1 -> Gain2/1
  PID Controller3/1 -> Out/1
  In/1 -> PID Controller3/1
  Constant4/1 -> PID Controller3/2

== system ROPOD_Control_WheelsRL_Code_GEN/RopodTorqueDistribution_/wheel vel cntr/Wheels Velocity controller/G_I_LL_LPF Controller6/Shapeit Integrator (Tustin) ==
  In : Inport
  I_fhz : Inport  Port=2
  reset : Inport  Port=3
  Constant : Constant  Value=0
  Constant4 : Constant
  Constant5 : Constant  Value=0
  Gain2 : Gain  Gain=2*pi
  PID Controller3 : pid_lib/PID Controller  Controller=PID  Form=Parallel  TimeDomain=Discrete-time  UseExternalTs=off  SampleTime=Ts  IntegratorMethod=Trapezoidal  FilterMethod=Trapezoidal  ControllerParametersSource=external  P=0.4  I=0.4*2*pi*3  D=0  UseFilter=on  N=100  TunerSelectOption=Transfer Function Based (PID Tuner App)  InitialConditionSource=internal  InitialConditionForIntegrator=0  InitialConditionForFilter=0  DifferentiatorICPrevScaledInput=0  ExternalReset=level  TrackingMode=off  Kt=1  LimitOutput=on  SatLimitsSource=internal  UpperSaturationLimit=max_hw_tau  LowerSaturationLimit=-max_hw_tau  LinearizeAsGain=on  AntiWindupMode=clamping  Kb=1  POutMin=[]  POutMax=[]  IOutMin=[]  IOutMax=[]  DOutMin=[]  DOutMax=[]  NOutMin=[]  NOutMax=[]  SumOutMin=[]  SumOutMax=[]  SaturationOutMin=[]  SaturationOutMax=[]  PParamMin=[]  PParamMax=[]  IParamMin=[]  IParamMax=[]  DParamMin=[]  DParamMax=[]  NParamMin=[]  NParamMax=[]  KbParamMin=[]  KbParamMax=[]  KtParamMin=[]  KtParamMax=[]  KbOutMin=[]  KbOutMax=[]  KtOutMin=[]  KtOutMax=[]  IntegratorOutMin=[]  IntegratorOutMax=[]  FilterOutMin=[]  FilterOutMax=[]  SumI1OutMin=[]  SumI1OutMax=[]  SumI2OutMin=[]  SumI2OutMax=[]  SumI3OutMin=[]  SumI3OutMax=[]  SumI4OutMin=[]  SumI4OutMax=[]  SumDOutMin=[]  SumDOutMax=[]  DifferentiatorOutMin=[]  DifferentiatorOutMax=[]  FilterDiffOutCoefMin=[]  FilterDiffOutCoefMax=[]  ReciprocalOutMin=[]  ReciprocalOutMax=[]  SumDenOutMin=[]  SumDenOutMax=[]  SumNumOutMin=[]  SumNumOutMax=[]  DivideOutMin=[]  DivideOutMax=[]  UdiffTsProdOutMin=[]  UdiffTsProdOutMax=[]  NTsProdOutMin=[]  NTsProdOutMax=[]  UintegralTsProdOutMin=[]  UintegralTsProdOutMax=[]  UngainTsProdOutMin=[]  UngainTsProdOutMax=[]  IntegratorContinuousStateAttributes=''  IntegratorStateMustResolveToSignalObject=off  IntegratorRTWStateStorageClass=Auto  FilterContinuousStateAttributes=''  FilterStateMustResolveToSignalObject=off  FilterRTWStateStorageClass=Auto  ParallelPVariant=ExternalParameters  IdealPVariant=Disabled  IVariant=ExternalParameters  DVariant=ExternalParameters  IntegratorVariant=Discrete  SatVariant=Enabled  AWVariant=DiscClampingParallel  PCopyVariant=Disabled  TRVariant=Disabled  FdbkBlocksVariant=Feedback  IdealPFdbkVariant=Passthrough  SatFdbkVariant=Passthrough  DerivativeFilterVariant=TrapezoidalFilter  NVariant=ExternalParameters  NCopyVariant=ExternalParameters  FilterICVariant=InternalICsFilter  IntegratorICVariant=InternalICs  ExternalResetVariant=ExternalReset  TRSumVariant=Passthrough  SumFdbkVariant=Enabled  SumVariant=Sum_PID  TsampFilterVariant=InternalTs  TsampNgainVariant=Passthrough  TsampIntegralVariant=Passthrough  ExternalSaturationOutDataTypeStr=Inherit: Same as second input
  Product4 : Product
  Out : Outport  VectorParamsAs1DForOutWhenUnconnected=off
  wires:
  I_fhz/1 -> Product4/2
  Product4/1 -> Gain2/1
  reset/1 -> PID Controller3/6
  Gain2/1 -> PID Controller3/3
  PID Controller3/1 -> Out/1
  In/1 -> PID Controller3/1
  Constant4/1 -> Product4/1, PID Controller3/2
  Constant5/1 -> PID Controller3/5
  Constant/1 -> PID Controller3/4

== system ROPOD_Control_WheelsRL_Code_GEN/RopodTorqueDistribution_/wheel vel cntr/Wheels Velocity controller/G_I_LL_LPF Controller6/Shapeit Lead-Lag (Tustin) ==
  In : Inport
  fz : Inport  Port=2
  fp : Inport  Port=3
  Add : Sum  Inputs=+-
  Constant1 : Constant
  Constant2 : Constant  Value=0
  Constant4 : Constant
  Divide : Product  Inputs=*/
  Divide1 : Product  Inputs=/*
  Gain1 : Gain  Gain=2*pi
  Gain2 : Gain  Gain=2*pi
  PID Controller3 : pid_lib/PID Controller  Controller=PID  Form=Parallel  TimeDomain=Discrete-time  UseExternalTs=off  SampleTime=Ts  IntegratorMethod=Trapezoidal  FilterMethod=Trapezoidal  ControllerParametersSource=external  P=0.4  I=0.4*2*pi*3  D=0  UseFilter=on  N=100  TunerSelectOption=Transfer Function Based (PID Tuner App)  InitialConditionSource=internal  InitialConditionForIntegrator=0  InitialConditionForFilter=0  DifferentiatorICPrevScaledInput=0  ExternalReset=none  TrackingMode=off  Kt=1  LimitOutput=off  SatLimitsSource=internal  UpperSaturationLimit=max_hw_tau  LowerSaturationLimit=-max_hw_tau  LinearizeAsGain=on  AntiWindupMode=clamping  Kb=1  POutMin=[]  POutMax=[]  IOutMin=[]  IOutMax=[]  DOutMin=[]  DOutMax=[]  NOutMin=[]  NOutMax=[]  SumOutMin=[]  SumOutMax=[]  SaturationOutMin=[]  SaturationOutMax=[]  PParamMin=[]  PParamMax=[]  IParamMin=[]  IParamMax=[]  DParamMin=[]  DParamMax=[]  NParamMin=[]  NParamMax=[]  KbParamMin=[]  KbParamMax=[]  KtParamMin=[]  KtParamMax=[]  KbOutMin=[]  KbOutMax=[]  KtOutMin=[]  KtOutMax=[]  IntegratorOutMin=[]  IntegratorOutMax=[]  FilterOutMin=[]  FilterOutMax=[]  SumI1OutMin=[]  SumI1OutMax=[]  SumI2OutMin=[]  SumI2OutMax=[]  SumI3OutMin=[]  SumI3OutMax=[]  SumI4OutMin=[]  SumI4OutMax=[]  SumDOutMin=[]  SumDOutMax=[]  DifferentiatorOutMin=[]  DifferentiatorOutMax=[]  FilterDiffOutCoefMin=[]  FilterDiffOutCoefMax=[]  ReciprocalOutMin=[]  ReciprocalOutMax=[]  SumDenOutMin=[]  SumDenOutMax=[]  SumNumOutMin=[]  SumNumOutMax=[]  DivideOutMin=[]  DivideOutMax=[]  UdiffTsProdOutMin=[]  UdiffTsProdOutMax=[]  NTsProdOutMin=[]  NTsProdOutMax=[]  UintegralTsProdOutMin=[]  UintegralTsProdOutMax=[]  UngainTsProdOutMin=[]  UngainTsProdOutMax=[]  IntegratorContinuousStateAttributes=''  IntegratorStateMustResolveToSignalObject=off  IntegratorRTWStateStorageClass=Auto  FilterContinuousStateAttributes=''  FilterStateMustResolveToSignalObject=off  FilterRTWStateStorageClass=Auto  ParallelPVariant=ExternalParameters  IdealPVariant=Disabled  IVariant=ExternalParameters  DVariant=ExternalParameters  IntegratorVariant=Discrete  SatVariant=Disabled  AWVariant=Passthrough  PCopyVariant=Disabled  TRVariant=Disabled  FdbkBlocksVariant=Forward  IdealPFdbkVariant=Disabled  SatFdbkVariant=Disabled  DerivativeFilterVariant=TrapezoidalFilter  NVariant=ExternalParameters  NCopyVariant=ExternalParameters  FilterICVariant=InternalICsFilter  IntegratorICVariant=InternalICs  ExternalResetVariant=Disabled  TRSumVariant=Passthrough  SumFdbkVariant=Disabled  SumVariant=Sum_PID  TsampFilterVariant=InternalTs  TsampNgainVariant=Passthrough  TsampIntegralVariant=Passthrough  ExternalSaturationOutDataTypeStr=Inherit: Same as second input
  Out : Outport  VectorParamsAs1DForOutWhenUnconnected=off
  wires:
  Constant4/1 -> PID Controller3/2
  In/1 -> PID Controller3/1
  PID Controller3/1 -> Out/1
  fz/1 -> Gain2/1
  fp/1 -> Gain1/1
  Gain1/1 -> PID Controller3/5, Divide/2
  Constant2/1 -> PID Controller3/3
  Gain2/1 -> Divide1/1, Divide/1
  Divide/1 -> Add/2
  Constant1/1 -> Add/1
  Add/1 -> Divide1/2
  Divide1/1 -> PID Controller3/4
